simulink model "OMSv1_2"  (Simulink 6.6)
settings: Solver=ode4  SolverMode=SingleTasking  StartTime=0.0  StopTime=5  FixedStep=0.001  MaxStep=0.001  RelTol=1e-3  AbsTol=1e-3
undefined symbols (not defined in the file): alexlaw, bs_onoff, bs_scale, bsfsacrit, bsfsvcrit, cnsgain, fs_onoff, fs_scale, fsdelaycalc, ltdrk, phasicgain, pmcgain, pmctau2, pmctau3, saccsw, spgain, tonicgain, tvrD, tvrN
(part 3 of 7)

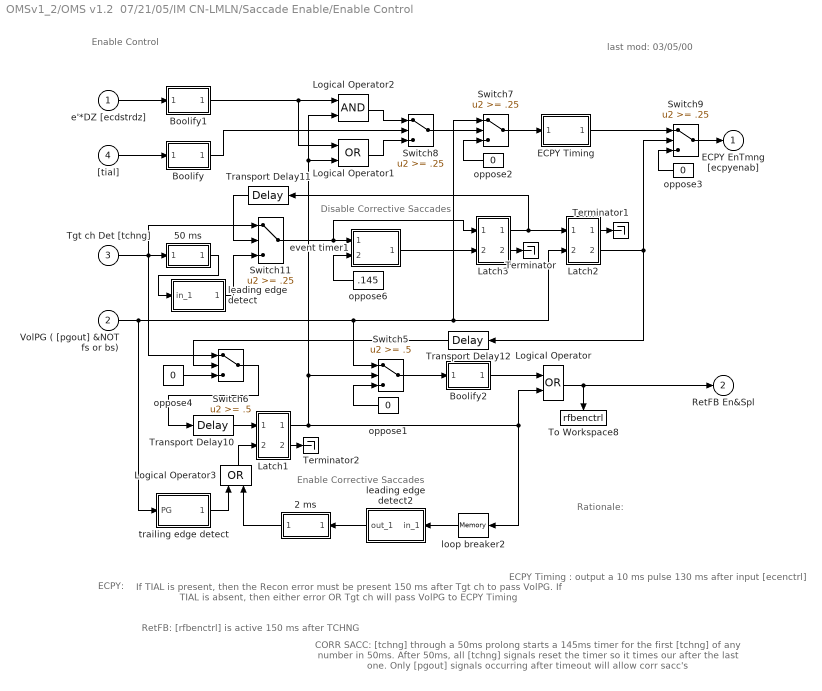
== system OMSv1_2/OMS v1.2  07/21/05/IM CN-LMLN/Saccade Enable/Enable Control ==
  note: Enable Control
  note: Enable
      | Corrective Saccades
  note: last mod:
      | 03/05/00
  note: Rationale:
  note: ECPY Timing : output a 10 ms pulse
      | 130 ms after input [ecenctrl]
  note: If TIAL is present, then the Recon error must be present 150 ms after Tgt ch to pass VolPG.
      | If TIAL is absent, then either error OR Tgt ch will pass VolPG to ECPY Timing
  note: ECPY:
  note: RetFB:
      | [rfbenctrl] is active 150 ms after TCHNG
  note: Disable
      | Corrective Saccades
  note: CORR SACC:
      | [tchng] through a 50ms prolong starts a 145ms timer for the
      | first [tchng] of any number in 50ms. After 50ms, all [tchng]
      | signals reset the timer so it times our after the last one.
      | Only [pgout] signals occurring after timeout will allow corr sacc's
  e'*DZ [ecdstrdz] : Inport
  VolPG ( [pgout] &NOT fs or bs) : Inport  Port=2
  Tgt ch Det [tchng] : Inport  Port=3
  "[tial]" : Inport  Port=4
  2 ms : Subsystem  Orientation=left  mask{prolong=2}
      mask prompts: prolong "Prolong pulse by?  (msec)"
      mask Display: disp('prolong')
  50 ms : Subsystem  mask{prolong=50}
      mask prompts: prolong "Prolong pulse by?  (msec)"
      mask Display: disp('prolong')
  Boolify : Subsystem
      mask Display: disp('Boolify')
  Boolify1 : Subsystem
      mask Display: disp('Boolify')
  Boolify2 : Subsystem
      mask Display: disp('Boolify')
  ECPY Timing : Subsystem
      mask Display: disp('ECPY\nTiming')
  Latch1 : Subsystem  mask(Latch){@1=0}
      mask prompts: @1 "Initial State for Output "Q":"
      mask help: Latch
      mask init:
      | ini=(@1~=0);
      mask Help: Latches the S input.  When S (set) is one, the Q output  becomes one.  The output remains one until the R (reset) input becomes one, forcing the output to zero.  If both R and S are one, the latch will be in an undefined state.
      mask Display: disp('S   Q\n\nR  !Q')
  Latch2 : Subsystem  mask(Latch){@1=0}
      mask prompts: @1 "Initial State for Output "Q":"
      mask help: Latch
      mask init:
      | ini=(@1~=0);
      mask Help: Latches the S input.  When S (set) is one, the Q output  becomes one.  The output remains one until the R (reset) input becomes one, forcing the output to zero.  If both R and S are one, the latch will be in an undefined state.
      mask Display: disp('S   Q\n\nR  !Q')
  Latch3 : Subsystem  mask(Latch){@1=0}
      mask prompts: @1 "Initial State for Output "Q":"
      mask help: Latch
      mask init:
      | ini=(@1~=0);
      mask Help: Latches the S input.  When S (set) is one, the Q output  becomes one.  The output remains one until the R (reset) input becomes one, forcing the output to zero.  If both R and S are one, the latch will be in an undefined state.
      mask Display: disp('S   Q\n\nR  !Q')
  Logical Operator : Logic  Operator=OR
  Logical Operator1 : Logic  Operator=OR
  Logical Operator2 : Logic
  Logical Operator3 : Logic  Orientation=up  Operator=OR
  Switch{7..9,11} (4 alike) : Switch  Threshold=.25  SaturateOnIntegerOverflow=on  InputSameDT=on
  Switch5 : Switch  Threshold=.5  SaturateOnIntegerOverflow=on  InputSameDT=on
  Switch6 : Switch  Threshold=.5  SaturateOnIntegerOverflow=on  InputSameDT=on
  Terminator : Terminator
  Terminator1 : Terminator
  Terminator2 : Terminator
  To Workspace8 : ToWorkspace  VariableName=rfbenctrl  SaveFormat=Array
      settings: Orientation=down  MaxDataPoints=10000
  Transport Delay10 : TransportDelay  DelayTime=.15
      mask Display: disp('150ms')
  Transport Delay11 : TransportDelay  Orientation=left  DelayTime=.05
      mask Display: disp('50ms')
  Transport Delay12 : TransportDelay  Orientation=left  DelayTime=.002
      mask Display: disp('2ms')
  event timer1 : Subsystem
      mask Display: disp('Event\nTimer2')
  leading edge detect : Subsystem
      mask Display: disp('Leading\nEdge Det')
  leading edge detect2 : Subsystem  Orientation=left
      mask Display: disp('Leading\nEdge Det')
  loop breaker2 : Memory  Orientation=left
  oppose1 : Constant  Orientation=left  Value=0
  oppose2 : Constant  Orientation=left  Value=0
  oppose3 : Constant  Orientation=left  Value=0
  oppose4 : Constant  Value=0
  oppose6 : Constant  Orientation=left  Value=.145
  trailing edge detect : Subsystem
      mask Display: disp('Trailing\nEdge Det')
  ECPY EnTmng [ecpyenab] : Outport  InitialOutput=0
  RetFB En&Spl : Outport  Port=2  InitialOutput=0
  wires:
  Boolify1/1(Out1) -> Logical Operator1/1, Logical Operator2/1
  "[tial]"/1 -> Boolify/1(In1)
  e'*DZ [ecdstrdz]/1 -> Boolify1/1(In1)
  Logical Operator1/1 -> Switch8/3
  Logical Operator2/1 -> Switch8/1
  Boolify/1(Out1) -> Switch8/2
  oppose2/1 -> Switch7/3
  Switch8/1 -> Switch7/2
  ECPY Timing/1(ECPY Enable [ecpyenab]) -> Switch9/1
  Switch9/1 -> ECPY EnTmng [ecpyenab]/1
  oppose3/1 -> Switch9/3
  Latch2/2(out_2) -> Transport Delay12/1, Switch9/2
  oppose6/1 -> event timer1/2(_timer value (port))
  Transport Delay11/1 -> Switch11/2
  Tgt ch Det [tchng]/1 -> 50 ms/1(value(in)), Switch6/1, Switch11/1
  Latch3/1(out_1) -> Latch2/1(in_1), Transport Delay11/1
  VolPG ( [pgout] &NOT fs or bs)/1 -> trailing edge detect/1(PG), Switch5/1, Switch7/1, Latch2/2(in_2)
  oppose1/1 -> Switch5/3
  Switch5/1 -> Boolify2/1(In1)
  Boolify2/1(Out1) -> Logical Operator/1
  Logical Operator/1 -> RetFB En&Spl/1, To Workspace8/1
  Latch1/1(out_1) -> Switch5/2, Logical Operator1/2, Logical Operator2/2, Logical Operator/2, loop breaker2/1
  Transport Delay10/1 -> Latch1/1(in_1)
  Logical Operator3/1 -> Latch1/2(in_2)
  oppose4/1 -> Switch6/3
  Switch6/1 -> Transport Delay10/1
  Transport Delay12/1 -> Switch6/2
  loop breaker2/1 -> leading edge detect2/1(in_1)
  50 ms/1(value(out)) -> leading edge detect/1(in_1)
  leading edge detect/1(out_1) -> Switch11/3
  Switch7/1 -> ECPY Timing/1(ECPY EnCntr [ecenctrl])
  event timer1/1(FF Reset) -> Latch3/2(in_2)
  Switch11/1 -> event timer1/1(SW out), Latch3/1(in_1)
  trailing edge detect/1(Latch R) -> Logical Operator3/1
  2 ms/1(value(out)) -> Logical Operator3/2
  leading edge detect2/1(out_1) -> 2 ms/1(value(in))
  Latch3/2(out_2) -> Terminator/1
  Latch2/1(out_1) -> Terminator1/1
  Latch1/2(out_2) -> Terminator2/1

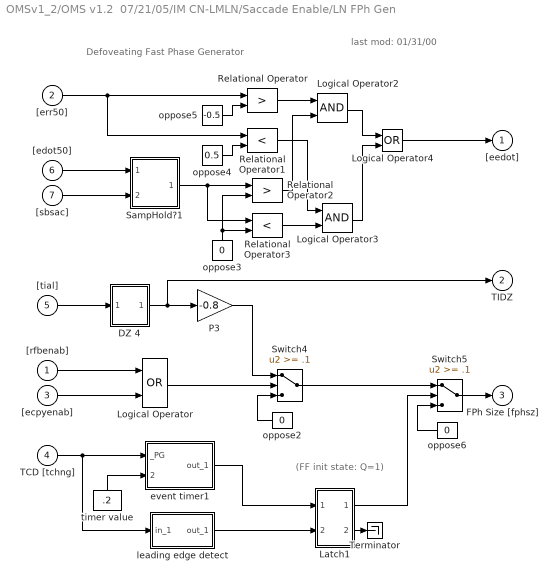
== system OMSv1_2/OMS v1.2  07/21/05/IM CN-LMLN/Saccade Enable/LN FPh Gen ==
  note: Defoveating Fast Phase Generator
  note: (FF init state: Q=1)
  note: last mod:
      | 01/31/00
  "[rfbenab]" : Inport
  "[err50]" : Inport  Port=2
  "[ecpyenab]" : Inport  Port=3
  TCD [tchng] : Inport  Port=4
  "[tial]" : Inport  Port=5
  "[edot50]" : Inport  Port=6
  "[sbsac]" : Inport  Port=7
  DZ 4 : Subsystem
      mask Display: disp('Dead\nZone')
  Latch1 : Subsystem  mask(Latch){@1=1}
      mask prompts: @1 "Initial State for Output "Q":"
      mask help: Latch
      mask init:
      | ini=(@1~=0);
      mask Help: Latches the S input.  When S (set) is one, the Q output  becomes one.  The output remains one until the R (reset) input becomes one, forcing the output to zero.  If both R and S are one, the latch will be in an undefined state.
      mask Display: disp('S   Q\n\nR  !Q')
  Logical Operator : Logic  Operator=OR
  Logical Operator2 : Logic
  Logical Operator3 : Logic
  Logical Operator4 : Logic  Operator=OR
  P3 : Gain  Gain=-0.8  SaturateOnIntegerOverflow=on
  Relational Operator : RelationalOperator  Operator=>  InputSameDT=on
  Relational Operator1 : RelationalOperator  Operator=<  InputSameDT=on
  Relational Operator2 : RelationalOperator  Operator=>  InputSameDT=on
  Relational Operator3 : RelationalOperator  Operator=<  InputSameDT=on
  SampHold?1 : Subsystem
      mask Display: disp('S&H\n(S=H)\n(H=L)')
  Switch4 : Switch  Threshold=.1  SaturateOnIntegerOverflow=on  InputSameDT=on
  Switch5 : Switch  Threshold=.1  SaturateOnIntegerOverflow=on  InputSameDT=on
  Terminator : Terminator
  event timer1 : Subsystem
      mask Display: disp('Event\nTimer2')
  leading edge detect : Subsystem
      mask Display: disp('Leading\nEdge Det')
  oppose2 : Constant  Orientation=left  Value=0
  oppose3 : Constant  Orientation=up  Value=0
  oppose4 : Constant  Value=0.5
  oppose5 : Constant  Value=-0.5
  oppose6 : Constant  Orientation=left  Value=0
  timer value : Constant  Orientation=up  Value=.2
  "[eedot]" : Outport  InitialOutput=0
  TIDZ : Outport  Port=2  InitialOutput=0
  FPh Size [fphsz] : Outport  Port=3  InitialOutput=0
  wires:
  "[err50]"/1 -> Relational Operator/1, Relational Operator1/1
  Logical Operator4/1 -> "[eedot]"/1
  Logical Operator2/1 -> Logical Operator4/1
  Relational Operator/1 -> Logical Operator2/1
  oppose5/1 -> Relational Operator/2
  oppose4/1 -> Relational Operator1/2
  Logical Operator3/1 -> Logical Operator4/2
  oppose3/1 -> Relational Operator3/2, Relational Operator2/2
  SampHold?1/1(output) -> Relational Operator2/1, Relational Operator3/1
  Relational Operator3/1 -> Logical Operator3/2
  Relational Operator2/1 -> Logical Operator2/2
  Relational Operator1/1 -> Logical Operator3/1
  "[sbsac]"/1 -> SampHold?1/2(S/H?)
  "[edot50]"/1 -> SampHold?1/1(Input)
  "[rfbenab]"/1 -> Logical Operator/1
  oppose2/1 -> Switch4/3
  "[ecpyenab]"/1 -> Logical Operator/2
  Switch4/1 -> Switch5/1
  Switch5/1 -> FPh Size [fphsz]/1
  oppose6/1 -> Switch5/3
  DZ 4/1(out_1) -> P3/1, TIDZ/1
  "[tial]"/1 -> DZ 4/1(in_1)
  event timer1/1(out_1) -> Latch1/1(in_1)
  leading edge detect/1(out_1) -> Latch1/2(in_2)
  Latch1/1(out_1) -> Switch5/2
  timer value/1 -> event timer1/2(_timer value (port))
  TCD [tchng]/1 -> event timer1/1(_PG), leading edge detect/1(in_1)
  P3/1 -> Switch4/1
  Logical Operator/1 -> Switch4/2
  Latch1/2(out_2) -> Terminator/1

== system OMSv1_2/OMS v1.2  07/21/05/IM CN-LMLN/Saccade Enable/Latch1 ==
  in_1 : Inport
  in_2 : Inport  Port=2
  Demux : Demux  Outputs=2
  Logic : CombinatorialLogic  TruthTable=[0 1;0 1;1 0;0 1;1 0;0 1;1 0;1 0]
  Memory : Memory  Orientation=left  X0=ini
  Mux : Mux  Inputs=3
  out_1 : Outport  InitialOutput=0
  out_2 : Outport  Port=2  InitialOutput=0
  wires:
  in_2/1 -> Mux/3
  in_1/1 -> Mux/2
  Memory/1 -> Mux/1
  Demux/1 -> Memory/1, out_1/1
  Mux/1 -> Logic/1
  Logic/1 -> Demux/1
  Demux/2 -> out_2/1

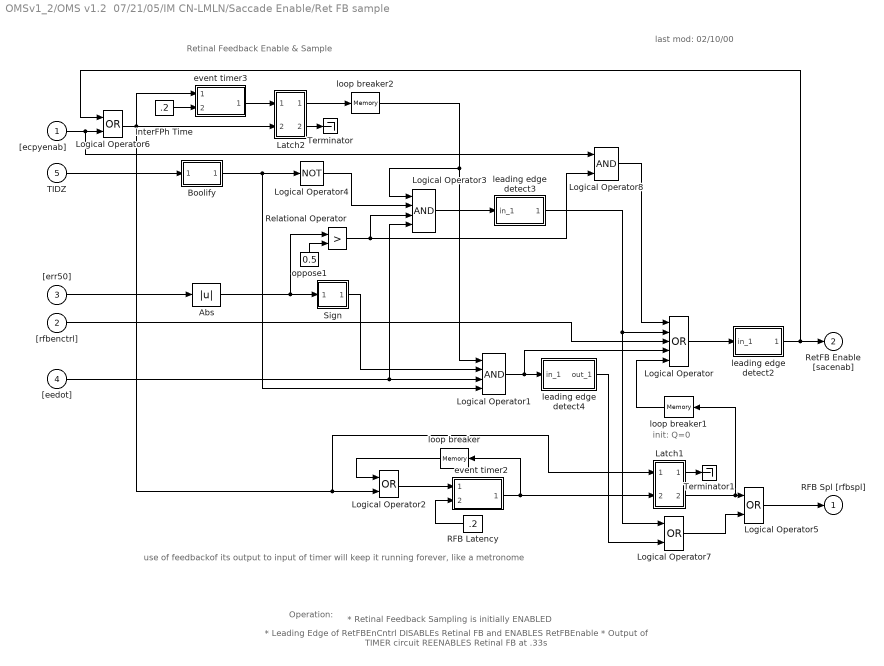
== system OMSv1_2/OMS v1.2  07/21/05/IM CN-LMLN/Saccade Enable/Ret FB sample ==
  note: * Leading Edge of RetFBEnCntrl DISABLEs Retinal FB
      |  and ENABLES RetFBEnable
      | * Output of TIMER circuit REENABLES Retinal FB at .33s
  note: * Retinal Feedback Sampling is initially ENABLED
  note: Operation:
  note: init: Q=0
  note: Retinal Feedback Enable & Sample
  note: last mod:
      | 02/10/00
  note: use of feedbackof its output to input of timer will
      | keep it running forever, like a metronome
  "[ecpyenab]" : Inport
  "[rfbenctrl]" : Inport  Port=2
  "[err50]" : Inport  Port=3
  "[eedot]" : Inport  Port=4
  TIDZ : Inport  Port=5
  Abs : Abs  SaturateOnIntegerOverflow=on
  Boolify : Subsystem
      mask Display: disp('Boolify')
  InterFPh Time : Constant  Value=.2
  Latch1 : Subsystem  mask(Latch){@1=0}
      mask prompts: @1 "Initial State for Output "Q":"
      mask help: Latch
      mask init:
      | ini=(@1~=0);
      mask Help: Latches the S input.  When S (set) is one, the Q output  becomes one.  The output remains one until the R (reset) input becomes one, forcing the output to zero.  If both R and S are one, the latch will be in an undefined state.
      mask Display: disp('S   Q\n\nR  !Q')
  Latch2 : Subsystem  mask(Latch){@1=1}
      mask prompts: @1 "Initial State for Output "Q":"
      mask help: Latch
      mask init:
      | ini=(@1~=0);
      mask Help: Latches the S input.  When S (set) is one, the Q output  becomes one.  The output remains one until the R (reset) input becomes one, forcing the output to zero.  If both R and S are one, the latch will be in an undefined state.
      mask Display: disp('S   Q\n\nR  !Q')
  Logical Operator : Logic  Operator=OR  Inputs=5
  Logical Operator1 : Logic  Inputs=4
  Logical Operator{2,5..7} (4 alike) : Logic  Operator=OR
  Logical Operator3 : Logic  Inputs=4
  Logical Operator4 : Logic  Operator=NOT  Inputs=1
  Logical Operator8 : Logic
  RFB Latency : Constant  Orientation=left  Value=.2
  Relational Operator : RelationalOperator  Operator=>  InputSameDT=on
  Sign : Subsystem
      mask Type: Sign
      mask Description: y = sign(x)
      mask Help: Sign Function:\n\t\t\ty = 1 if x > 0\n\t\t\ty = 0 if x = 0\n\t\t\ty = -1 if x < 0
      mask Display: plot(-50,-50,50,50,[-50,50],[0,0],[0,0],[-50,50],[-40,0],[-30,-30],[0,40],[30,30])
  Terminator : Terminator
  Terminator1 : Terminator
  event timer2 : Subsystem
      mask Display: disp('Event\nTimer2')
  event timer3 : Subsystem
      mask Display: disp('Event\nTimer2')
  leading edge detect2 : Subsystem
      mask Display: disp('Leading\nEdge Det')
  leading edge detect3 : Subsystem
      mask Display: disp('Leading\nEdge Det')
  leading edge detect4 : Subsystem
      mask Display: disp('Leading\nEdge Det')
  loop breaker : Memory  Orientation=left
  loop breaker1 : Memory  Orientation=left
  loop breaker2 : Memory
  oppose1 : Constant  Orientation=up  Value=0.5
  RFB Spl [rfbspl] : Outport  InitialOutput=0
  RetFB Enable [sacenab] : Outport  Port=2  InitialOutput=0
  wires:
  InterFPh Time/1 -> event timer3/2(_timer value (port))
  event timer3/1(outFF) -> Latch2/1(in_1)
  Latch2/1(out_1) -> loop breaker2/1
  Boolify/1(Out1) -> Logical Operator4/1, Logical Operator1/4
  TIDZ/1 -> Boolify/1(In1)
  loop breaker/1 -> Logical Operator2/1
  RFB Latency/1 -> event timer2/2(_timer value (port))
  oppose1/1 -> Relational Operator/2
  Abs/1 -> Sign/1(in_1), Relational Operator/1
  Logical Operator6/1 -> event timer3/1(RetFB EnCntrl), Latch2/2(in_2), Logical Operator2/2, Latch1/1(in_1)
  Logical Operator3/1 -> leading edge detect3/1(in_1)
  leading edge detect2/1(out_1) -> Logical Operator6/1, RetFB Enable [sacenab]/1
  Logical Operator1/1 -> leading edge detect4/1(in_1), Logical Operator/4
  leading edge detect4/1(out_1) -> Logical Operator7/2
  "[ecpyenab]"/1 -> Logical Operator6/2, Logical Operator8/1
  loop breaker1/1 -> Logical Operator/5
  "[rfbenctrl]"/1 -> Logical Operator/3
  leading edge detect3/1(out_1) -> Logical Operator7/1, Logical Operator/2
  event timer2/1(outFF) -> Latch1/2(in_2), loop breaker/1
  "[eedot]"/1 -> Logical Operator1/3, Logical Operator3/4
  Latch1/2(out_2) -> loop breaker1/1, Logical Operator5/1
  Logical Operator5/1 -> RFB Spl [rfbspl]/1
  Relational Operator/1 -> Logical Operator3/3, Logical Operator8/2
  Sign/1(out_1) -> Logical Operator1/2
  "[err50]"/1 -> Abs/1
  loop breaker2/1 -> Logical Operator1/1, Logical Operator3/1
  Logical Operator8/1 -> Logical Operator/1
  Logical Operator7/1 -> Logical Operator5/2
  Logical Operator2/1 -> event timer2/1(RetFB EnCntrl)
  Logical Operator4/1 -> Logical Operator3/2
  Logical Operator/1 -> leading edge detect2/1(in_1)
  Latch2/2(out_2) -> Terminator/1
  Latch1/1(out_1) -> Terminator1/1

== system OMSv1_2/OMS v1.2  07/21/05/IM CN-LMLN/Saccade Enable/leading edge detect2 ==
  note: It is also possible to remove the SIGNUM function
      | and the '==', and replace them with a simple
      | switch with a threshold of (say) 150 or so.
  note: leading edge detection
  in_1 : Inport
  Abs : Abs  SaturateOnIntegerOverflow=on
  Derivative : Derivative
  Relational Operator : RelationalOperator  Operator===  InputSameDT=on
  Sign : Subsystem
      mask Type: Sign
      mask Description: y = sign(x)
      mask Help: Sign Function:\n\t\t\ty = 1 if x > 0\n\t\t\ty = 0 if x = 0\n\t\t\ty = -1 if x < 0
      mask Display: plot(-50,-50,50,50,[-50,50],[0,0],[0,0],[-50,50],[-40,0],[-30,-30],[0,40],[30,30])
  Threshold 1 : Constant
  out_1 : Outport  InitialOutput=0
  wires:
  Abs/1 -> Derivative/1
  Derivative/1 -> Sign/1(in_1)
  Sign/1(out_1) -> Relational Operator/1
  Threshold 1/1 -> Relational Operator/2
  Relational Operator/1 -> out_1/1
  in_1/1 -> Abs/1

== system OMSv1_2/OMS v1.2  07/21/05/IM CN-LMLN/Saccade Enable/prolong ==
  note: init Q = 0
  note: Stretch the duration of an input pulse, latching it at its value at pulse onset.
  note: The one integration step delay before the S&H block's S/H (bottom) input insures
      | that the input value to be latched is available to theS&H block's top input
      | before the S&H block tries to 'hold'.
  note: The start of the input pulse causes the value on input 1 to be held starting when the leading
      | edge occurs, and this value remains latched until 'delay' seconds after the pulse ends (trailing edge).
  note: 11/22/99
  note: init = 0
  note: init = 0
  value(in) : Inport
  " x/1000" : Constant  Orientation=up  Value=0.001
  Latch1 : Subsystem  mask(Latch){@1=0}
      mask prompts: @1 "Initial State for Output "Q":"
      mask help: Latch
      mask init:
      | ini=(@1~=0);
      mask Help: Latches the S input.  When S (set) is one, the Q output  becomes one.  The output remains one until the R (reset) input becomes one, forcing the output to zero.  If both R and S are one, the latch will be in an undefined state.
      mask Display: disp('S   Q\n\nR  !Q')
  Product : Product  SaturateOnIntegerOverflow=on  RndMeth=Zero  InputSameDT=on
  SampHold?2 : Subsystem
      mask Display: disp('S=L\nH=H')
  Terminator : Terminator
  Variable Transport Delay : VariableTransportDelay  MaximumDelay=10  MaximumPoints=prolong_buffersize
  leading edge detect : Subsystem
      mask Display: disp('Leading\nEdge Det')
  loop breaker2 : Memory
  stretch : Constant  Value=prolong
  trailing edge detect : Subsystem
      mask Display: disp('Trailing\nEdge Det')
  value(out) : Outport  InitialOutput=0
  wires:
  value(in)/1 -> leading edge detect/1(in_1), trailing edge detect/1(in_1), SampHold?2/1(Input)
  Variable Transport Delay/1 -> Latch1/2(in_2)
  trailing edge detect/1(out_1) -> Variable Transport Delay/1
  leading edge detect/1(out_1) -> Latch1/1(in_1)
  Latch1/1(out_1) -> loop breaker2/1
  SampHold?2/1(output) -> value(out)/1
  loop breaker2/1 -> SampHold?2/2(S/H?)
  stretch/1 -> Product/1
  Product/1 -> Variable Transport Delay/2
  " x/1000"/1 -> Product/2
  Latch1/2(out_2) -> Terminator/1

== system OMSv1_2/OMS v1.2  07/21/05/IM CN-LMLN/Saccade Enable/trailing edge detect ==
  note: trailing edge detection
  note: It is also possible to remove the SIGNUM function
      | and the '==', and replace them with a simple
      | switch with a threshold of (say) 150 or so.
  PG : Inport
  Abs : Abs  SaturateOnIntegerOverflow=on
  Derivative : Derivative
  Relational Operator : RelationalOperator  Operator===  InputSameDT=on
  Sign : Subsystem
      mask Type: Sign
      mask Description: y = sign(x)
      mask Help: Sign Function:\n\t\t\ty = 1 if x > 0\n\t\t\ty = 0 if x = 0\n\t\t\ty = -1 if x < 0
      mask Display: plot(-50,-50,50,50,[-50,50],[0,0],[0,0],[-50,50],[-40,0],[-30,-30],[0,40],[30,30])
  Threshold 1 : Constant  Value=-1
  Latch R : Outport  InitialOutput=0
  wires:
  PG/1 -> Abs/1
  Relational Operator/1 -> Latch R/1
  Threshold 1/1 -> Relational Operator/2
  Sign/1(out_1) -> Relational Operator/1
  Derivative/1 -> Sign/1(in_1)
  Abs/1 -> Derivative/1

== system OMSv1_2/OMS v1.2  07/21/05/IM CN-LMLN/Saccade Motor Commmand/TCHNG Override ==
  note: (FF init state: Q=1)
  note: * Leading Edge of input ENABLEs output
  note: Operation:
  note: *FS Enabling is initially DISABLED
  note: * Output of TIMER circuit DISABLES output
  note: TCHNG Override
  "[tchng]" : Inport
  timer dur : Inport  Orientation=up  Port=2
  Latch1 : Subsystem  mask(Latch){@1=1}
      mask prompts: @1 "Initial State for Output "Q":"
      mask help: Latch
      mask init:
      | ini=(@1~=0);
      mask Help: Latches the S input.  When S (set) is one, the Q output  becomes one.  The output remains one until the R (reset) input becomes one, forcing the output to zero.  If both R and S are one, the latch will be in an undefined state.
      mask Display: disp('S   Q\n\nR  !Q')
  Terminator : Terminator
  event timer2 : Subsystem
      mask Display: disp('Event\nTimer2')
  leading edge detect : Subsystem
      mask Display: disp('Leading\nEdge Det')
  tchng sw : Outport  InitialOutput=0
  wires:
  "[tchng]"/1 -> leading edge detect/1(in_1), event timer2/1(_PG)
  timer dur/1 -> event timer2/2(_timer value (port))
  event timer2/1(out_1) -> Latch1/1(in_1)
  leading edge detect/1(out_1) -> Latch1/2(in_2)
  Latch1/1(out_1) -> tchng sw/1
  Latch1/2(out_2) -> Terminator/1

== system OMSv1_2/OMS v1.2  07/21/05/IM CN-LMLN/Saccade Motor Commmand/Voluntary Saccade Switch ==
  note: Voluntary Saccade Switch
  note: move this outpt
      | to top switch
  note: last mod:
      | 02/26/01
  "[fphmag]" : Inport
  "[sacenab]" : Inport  Port=2
  "[fsorbs30]" : Inport  Port=3
  (0.5)1 : Switch  Threshold=.5  SaturateOnIntegerOverflow=on  InputSameDT=on
  (0.5)2 : Switch  Threshold=.5  SaturateOnIntegerOverflow=on  InputSameDT=on
  (0.5)3 : Switch  Threshold=.5  SaturateOnIntegerOverflow=on  InputSameDT=on
  Logical Operator4 : Logic  Operator=NOT  Inputs=1
  Logical Operator6 : Logic  Operator=OR
  oppose3 : Constant  Orientation=left  Value=0
  saccsw : Constant  Orientation=left  Value=saccsw
  "[vsmc]" : Outport  InitialOutput=0
  sacenab/0 : Outport  Port=2  InitialOutput=0
  wires:
  "[fphmag]"/1 -> (0.5)2/1
  "[fsorbs30]"/1 -> Logical Operator4/1
  Logical Operator4/1 -> Logical Operator6/2
  (0.5)2/1 -> (0.5)3/1
  Logical Operator6/1 -> sacenab/0/1
  saccsw/1 -> (0.5)2/3, (0.5)2/2, (0.5)1/2, (0.5)1/3
  "[sacenab]"/1 -> (0.5)1/1, (0.5)3/2
  (0.5)1/1 -> Logical Operator6/1
  oppose3/1 -> (0.5)3/3
  (0.5)3/1 -> "[vsmc]"/1

== system OMSv1_2/OMS v1.2  07/21/05/IM CN-LMLN/Sampled Target Reconstruction/Boolify ==
  In1 : Inport
  Abs2 : Abs  SaturateOnIntegerOverflow=on
  direction1 : Subsystem
      mask Type: Sign
      mask Description: y = sign(x)
      mask Help: Sign Function:\n\t\t\ty = 1 if x > 0\n\t\t\ty = 0 if x = 0\n\t\t\ty = -1 if x < 0
      mask Display: plot(-50,-50,50,50,[-50,50],[0,0],[0,0],[-50,50],[-40,0],[-30,-30],[0,40],[30,30])
  Out1 : Outport  InitialOutput=0
  wires:
  direction1/1(out_1) -> Out1/1
  In1/1 -> Abs2/1
  Abs2/1 -> direction1/1(in_1)

== system OMSv1_2/OMS v1.2  07/21/05/IM CN-LMLN/Sampled Target Reconstruction/Boolify1 ==
  In1 : Inport
  Abs2 : Abs  SaturateOnIntegerOverflow=on
  direction1 : Subsystem
      mask Type: Sign
      mask Description: y = sign(x)
      mask Help: Sign Function:\n\t\t\ty = 1 if x > 0\n\t\t\ty = 0 if x = 0\n\t\t\ty = -1 if x < 0
      mask Display: plot(-50,-50,50,50,[-50,50],[0,0],[0,0],[-50,50],[-40,0],[-30,-30],[0,40],[30,30])
  Out1 : Outport  InitialOutput=0
  wires:
  Abs2/1 -> direction1/1(in_1)
  In1/1 -> Abs2/1
  direction1/1(out_1) -> Out1/1

== system OMSv1_2/OMS v1.2  07/21/05/IM CN-LMLN/Sampled Target Reconstruction/DZ 0.3 ==
  note: We just output zero when the dead zone is in effect, and leave the
      |  output alone the rest of the time.
  note: This block is a better implementation of a dead zone than  the
      | block supplied by SIMULINK, because here we don't _subtract_
      | the dead zone from the rest of output.
  in_1 : Inport
  Abs : Abs  Orientation=down  SaturateOnIntegerOverflow=on
  Relational Operator : RelationalOperator  InputSameDT=on
  Switch6 : Switch  Threshold=.5  SaturateOnIntegerOverflow=on  InputSameDT=on
  dead zone : Constant  Orientation=up  Value=.3
  pos (deg) criterion1 : Constant  Orientation=left  Value=0
  out_1 : Outport  InitialOutput=0
  wires:
  Relational Operator/1 -> Switch6/2
  dead zone/1 -> Relational Operator/2
  pos (deg) criterion1/1 -> Switch6/3
  Abs/1 -> Relational Operator/1
  in_1/1 -> Abs/1, Switch6/1
  Switch6/1 -> out_1/1

== system OMSv1_2/OMS v1.2  07/21/05/IM CN-LMLN/Sampled Target Reconstruction/Latch1 ==
  in_1 : Inport
  in_2 : Inport  Port=2
  Demux : Demux  Outputs=2
  Logic : CombinatorialLogic  TruthTable=[0 1;0 1;1 0;0 1;1 0;0 1;1 0;1 0]
  Memory : Memory  Orientation=left  X0=ini
  Mux : Mux  Inputs=3
  out_1 : Outport  InitialOutput=0
  out_2 : Outport  Port=2  InitialOutput=0
  wires:
  in_2/1 -> Mux/3
  in_1/1 -> Mux/2
  Memory/1 -> Mux/1
  Demux/1 -> out_1/1, Memory/1
  Mux/1 -> Logic/1
  Logic/1 -> Demux/1
  Demux/2 -> out_2/1

== system OMSv1_2/OMS v1.2  07/21/05/IM CN-LMLN/Sampled Target Reconstruction/Latch2 ==
  in_1 : Inport
  in_2 : Inport  Port=2
  Demux : Demux  Outputs=2
  Logic : CombinatorialLogic  TruthTable=[0 1;0 1;1 0;0 1;1 0;0 1;1 0;1 0]
  Memory : Memory  Orientation=left  X0=ini
  Mux : Mux  Inputs=3
  out_1 : Outport  InitialOutput=0
  out_2 : Outport  Port=2  InitialOutput=0
  wires:
  Demux/2 -> out_2/1
  Logic/1 -> Demux/1
  Mux/1 -> Logic/1
  Demux/1 -> Memory/1, out_1/1
  Memory/1 -> Mux/1
  in_1/1 -> Mux/2
  in_2/1 -> Mux/3

== system OMSv1_2/OMS v1.2  07/21/05/IM CN-LMLN/Sampled Target Reconstruction/SampHold? ==
  note: When "S/H?" is HIGH, then "Input" is switched directly to the
      | output ("sample").  When "S/H?" is LOW, the current output is
      | maintained ("hold").
  Input : Inport
  S/H? : Inport  Port=2
  Memory : Memory  Orientation=left
  Sign : Subsystem
      mask Type: Sign
      mask Description: y = sign(x)
      mask Help: Sign Function:\n\t\t\ty = 1 if x > 0\n\t\t\ty = 0 if x = 0\n\t\t\ty = -1 if x < 0
      mask Display: plot(-50,-50,50,50,[-50,50],[0,0],[0,0],[-50,50],[-40,0],[-30,-30],[0,40],[30,30])
  Switch2 : Switch  Threshold=0.5  SaturateOnIntegerOverflow=on  InputSameDT=on
  output : Outport  InitialOutput=0
  wires:
  S/H?/1 -> Sign/1(in_1)
  Sign/1(out_1) -> Switch2/2
  Input/1 -> Switch2/1
  Switch2/1 -> output/1, Memory/1
  Memory/1 -> Switch2/3

== system OMSv1_2/OMS v1.2  07/21/05/IM CN-LMLN/Sampled Target Reconstruction/leading edge detect1 ==
  note: leading edge detection
  in_1 : Inport
  Abs : Abs  SaturateOnIntegerOverflow=on
  Derivative : Derivative
  Relational Operator : RelationalOperator  Operator===  InputSameDT=on
  Sign : Subsystem
      mask Type: Sign
      mask Description: y = sign(x)
      mask Help: Sign Function:\n\t\t\ty = 1 if x > 0\n\t\t\ty = 0 if x = 0\n\t\t\ty = -1 if x < 0
      mask Display: plot(-50,-50,50,50,[-50,50],[0,0],[0,0],[-50,50],[-40,0],[-30,-30],[0,40],[30,30])
  Threshold 1 : Constant
  out_1 : Outport  InitialOutput=0
  wires:
  Abs/1 -> Derivative/1
  Derivative/1 -> Sign/1(in_1)
  Sign/1(out_1) -> Relational Operator/1
  Threshold 1/1 -> Relational Operator/2
  Relational Operator/1 -> out_1/1
  in_1/1 -> Abs/1

== system OMSv1_2/OMS v1.2  07/21/05/IM CN-LMLN/Sampled Target Reconstruction/leading edge detect2 ==
  note: leading edge detection
  in_1 : Inport
  Abs : Abs  SaturateOnIntegerOverflow=on
  Derivative : Derivative
  Relational Operator : RelationalOperator  Operator===  InputSameDT=on
  Sign : Subsystem
      mask Type: Sign
      mask Description: y = sign(x)
      mask Help: Sign Function:\n\t\t\ty = 1 if x > 0\n\t\t\ty = 0 if x = 0\n\t\t\ty = -1 if x < 0
      mask Display: plot(-50,-50,50,50,[-50,50],[0,0],[0,0],[-50,50],[-40,0],[-30,-30],[0,40],[30,30])
  Threshold 1 : Constant
  out_1 : Outport  InitialOutput=0
  wires:
  in_1/1 -> Abs/1
  Relational Operator/1 -> out_1/1
  Threshold 1/1 -> Relational Operator/2
  Sign/1(out_1) -> Relational Operator/1
  Derivative/1 -> Sign/1(in_1)
  Abs/1 -> Derivative/1

== system OMSv1_2/OMS v1.2  07/21/05/IM CN-LMLN/Sampled Target Reconstruction/prolong ==
  note: init = 0
  note: init = 0
  note: 11/22/99
  note: The start of the input pulse causes the value on input 1 to be held starting when the leading
      | edge occurs, and this value remains latched until 'delay' seconds after the pulse ends (trailing edge).
  note: The one integration step delay before the S&H block's S/H (bottom) input insures
      | that the input value to be latched is available to theS&H block's top input
      | before the S&H block tries to 'hold'.
  note: Stretch the duration of an input pulse, latching it at its value at pulse onset.
  note: init Q = 0
  value(in) : Inport
  " x/1000" : Constant  Orientation=up  Value=0.001
  Latch1 : Subsystem  mask(Latch){@1=0}
      mask prompts: @1 "Initial State for Output "Q":"
      mask help: Latch
      mask init:
      | ini=(@1~=0);
      mask Help: Latches the S input.  When S (set) is one, the Q output  becomes one.  The output remains one until the R (reset) input becomes one, forcing the output to zero.  If both R and S are one, the latch will be in an undefined state.
      mask Display: disp('S   Q\n\nR  !Q')
  Product : Product  SaturateOnIntegerOverflow=on  RndMeth=Zero  InputSameDT=on
  SampHold?2 : Subsystem
      mask Display: disp('S=L\nH=H')
  Terminator : Terminator
  Variable Transport Delay : VariableTransportDelay  MaximumDelay=10  MaximumPoints=prolong_buffersize
  leading edge detect : Subsystem
      mask Display: disp('Leading\nEdge Det')
  loop breaker2 : Memory
  stretch : Constant  Value=prolong
  trailing edge detect : Subsystem
      mask Display: disp('Trailing\nEdge Det')
  value(out) : Outport  InitialOutput=0
  wires:
  " x/1000"/1 -> Product/2
  Product/1 -> Variable Transport Delay/2
  stretch/1 -> Product/1
  loop breaker2/1 -> SampHold?2/2(S/H?)
  SampHold?2/1(output) -> value(out)/1
  Latch1/1(out_1) -> loop breaker2/1
  leading edge detect/1(out_1) -> Latch1/1(in_1)
  trailing edge detect/1(out_1) -> Variable Transport Delay/1
  Variable Transport Delay/1 -> Latch1/2(in_2)
  value(in)/1 -> SampHold?2/1(Input), trailing edge detect/1(in_1), leading edge detect/1(in_1)
  Latch1/2(out_2) -> Terminator/1

== system OMSv1_2/OMS v1.2  07/21/05/IM CN-LMLN/Sampled Target Reconstruction/prolong1 ==
  note: init Q = 0
  note: Stretch the duration of an input pulse, latching it at its value at pulse onset.
  note: The one integration step delay before the S&H block's S/H (bottom) input insures
      | that the input value to be latched is available to theS&H block's top input
      | before the S&H block tries to 'hold'.
  note: The start of the input pulse causes the value on input 1 to be held starting when the leading
      | edge occurs, and this value remains latched until 'delay' seconds after the pulse ends (trailing edge).
  note: 11/22/99
  note: init = 0
  note: init = 0
  value(in) : Inport
  " x/1000" : Constant  Orientation=up  Value=0.001
  Latch1 : Subsystem  mask(Latch){@1=0}
      mask prompts: @1 "Initial State for Output "Q":"
      mask help: Latch
      mask init:
      | ini=(@1~=0);
      mask Help: Latches the S input.  When S (set) is one, the Q output  becomes one.  The output remains one until the R (reset) input becomes one, forcing the output to zero.  If both R and S are one, the latch will be in an undefined state.
      mask Display: disp('S   Q\n\nR  !Q')
  Product : Product  SaturateOnIntegerOverflow=on  RndMeth=Zero  InputSameDT=on
  SampHold?2 : Subsystem
      mask Display: disp('S=L\nH=H')
  Terminator : Terminator
  Variable Transport Delay : VariableTransportDelay  MaximumDelay=10  MaximumPoints=prolong_buffersize
  leading edge detect : Subsystem
      mask Display: disp('Leading\nEdge Det')
  loop breaker2 : Memory
  stretch : Constant  Value=prolong
  trailing edge detect : Subsystem
      mask Display: disp('Trailing\nEdge Det')
  value(out) : Outport  InitialOutput=0
  wires:
  value(in)/1 -> leading edge detect/1(in_1), trailing edge detect/1(in_1), SampHold?2/1(Input)
  Variable Transport Delay/1 -> Latch1/2(in_2)
  trailing edge detect/1(out_1) -> Variable Transport Delay/1
  leading edge detect/1(out_1) -> Latch1/1(in_1)
  Latch1/1(out_1) -> loop breaker2/1
  SampHold?2/1(output) -> value(out)/1
  loop breaker2/1 -> SampHold?2/2(S/H?)
  stretch/1 -> Product/1
  Product/1 -> Variable Transport Delay/2
  " x/1000"/1 -> Product/2
  Latch1/2(out_2) -> Terminator/1

== system OMSv1_2/OMS v1.2  07/21/05/IM CN-LMLN/Sampled Target Reconstruction/prolong2 ==
  note: init = 0
  note: init = 0
  note: 11/22/99
  note: The start of the input pulse causes the value on input 1 to be held starting when the leading
      | edge occurs, and this value remains latched until 'delay' seconds after the pulse ends (trailing edge).
  note: The one integration step delay before the S&H block's S/H (bottom) input insures
      | that the input value to be latched is available to theS&H block's top input
      | before the S&H block tries to 'hold'.
  note: Stretch the duration of an input pulse, latching it at its value at pulse onset.
  note: init Q = 0
  value(in) : Inport
  " x/1000" : Constant  Orientation=up  Value=0.001
  Latch1 : Subsystem  mask(Latch){@1=0}
      mask prompts: @1 "Initial State for Output "Q":"
      mask help: Latch
      mask init:
      | ini=(@1~=0);
      mask Help: Latches the S input.  When S (set) is one, the Q output  becomes one.  The output remains one until the R (reset) input becomes one, forcing the output to zero.  If both R and S are one, the latch will be in an undefined state.
      mask Display: disp('S   Q\n\nR  !Q')
  Product : Product  SaturateOnIntegerOverflow=on  RndMeth=Zero  InputSameDT=on
  SampHold?2 : Subsystem
      mask Display: disp('S=L\nH=H')
  Terminator : Terminator
  Variable Transport Delay : VariableTransportDelay  MaximumDelay=10  MaximumPoints=prolong_buffersize
  leading edge detect : Subsystem
      mask Display: disp('Leading\nEdge Det')
  loop breaker2 : Memory
  stretch : Constant  Value=prolong
  trailing edge detect : Subsystem
      mask Display: disp('Trailing\nEdge Det')
  value(out) : Outport  InitialOutput=0
  wires:
  " x/1000"/1 -> Product/2
  Product/1 -> Variable Transport Delay/2
  stretch/1 -> Product/1
  loop breaker2/1 -> SampHold?2/2(S/H?)
  SampHold?2/1(output) -> value(out)/1
  Latch1/1(out_1) -> loop breaker2/1
  leading edge detect/1(out_1) -> Latch1/1(in_1)
  trailing edge detect/1(out_1) -> Variable Transport Delay/1
  Variable Transport Delay/1 -> Latch1/2(in_2)
  value(in)/1 -> SampHold?2/1(Input), trailing edge detect/1(in_1), leading edge detect/1(in_1)
  Latch1/2(out_2) -> Terminator/1

== system OMSv1_2/OMS v1.2  07/21/05/IM CN-LMLN/Slip Velocity Reconstruction/DZ 0.5 ==
  note: We just output zero when the dead zone is in effect, and leave the
      |  output alone the rest of the time.
  note: This block is a better implementation of a dead zone than  the
      | block supplied by SIMULINK, because here we don't _subtract_
      | the dead zone from the rest of output.
  in_1 : Inport
  in_2 : Inport  Port=2
  Abs : Abs  Orientation=down  SaturateOnIntegerOverflow=on
  Relational Operator : RelationalOperator  InputSameDT=on
  Switch6 : Switch  Threshold=.5  SaturateOnIntegerOverflow=on  InputSameDT=on
  pos (deg) criterion1 : Constant  Orientation=left  Value=0
  out_1 : Outport  InitialOutput=0
  wires:
  Relational Operator/1 -> Switch6/2
  pos (deg) criterion1/1 -> Switch6/3
  Switch6/1 -> out_1/1
  in_2/1 -> Relational Operator/2
  Abs/1 -> Relational Operator/1
  in_1/1 -> Abs/1, Switch6/1

== system OMSv1_2/OMS v1.2  07/21/05/IM CN-LMLN/Slip Velocity Reconstruction/Lim 100 ==
  note: This block limits outputs to less than or equal to the "Limit" constant.
      | Inputs greater than "Limit" yield a zero output.
  in_1 : Inport
  Abs : Abs  SaturateOnIntegerOverflow=on
  Limit : Constant  Orientation=up  Value=100
  Product : Product  SaturateOnIntegerOverflow=on  RndMeth=Zero  InputSameDT=on
  Relational Operator : RelationalOperator  Operator=<=  InputSameDT=on
  out_1 : Outport  InitialOutput=0
  wires:
  in_1/1 -> Product/1, Abs/1
  Abs/1 -> Relational Operator/1
  Relational Operator/1 -> Product/2
  Limit/1 -> Relational Operator/2
  Product/1 -> out_1/1

== system OMSv1_2/OMS v1.2  07/21/05/IM CN-LMLN/Slip Velocity Reconstruction/SampHold?4 ==
  note: When "S/H?" is HIGH, then "Input" is switched directly to the
      | output ("sample").  When "S/H?" is LOW, the current output is
      | maintained ("hold").
  Input : Inport
  S/H? : Inport  Port=2
  Memory : Memory  Orientation=left
  Sign : Subsystem
      mask Type: Sign
      mask Description: y = sign(x)
      mask Help: Sign Function:\n\t\t\ty = 1 if x > 0\n\t\t\ty = 0 if x = 0\n\t\t\ty = -1 if x < 0
      mask Display: plot(-50,-50,50,50,[-50,50],[0,0],[0,0],[-50,50],[-40,0],[-30,-30],[0,40],[30,30])
  Switch2 : Switch  Threshold=0.5  SaturateOnIntegerOverflow=on  InputSameDT=on
  output : Outport  InitialOutput=0
  wires:
  S/H?/1 -> Sign/1(in_1)
  Sign/1(out_1) -> Switch2/2
  Switch2/1 -> output/1, Memory/1
  Input/1 -> Switch2/1
  Memory/1 -> Switch2/3

== system OMSv1_2/OMS v1.2  07/21/05/OMN2/SampHold?/Sign ==
  in_1 : Inport
  Constant : Constant  Value=0
  Relational Operator : RelationalOperator  Operator=>  InputSameDT=on
  Relational Operator1 : RelationalOperator  Operator=<  InputSameDT=on
  Sum : Sum  Inputs=+-  SaturateOnIntegerOverflow=on  InputSameDT=on
  out_1 : Outport  InitialOutput=0
  wires:
  in_1/1 -> Relational Operator/1, Relational Operator1/1
  Constant/1 -> Relational Operator1/2, Relational Operator/2
  Relational Operator1/1 -> Sum/2
  Relational Operator/1 -> Sum/1
  Sum/1 -> out_1/1

== system OMSv1_2/OMS v1.2  07/21/05/PG w rNI1/PW funct/Good Reset Integrator1 ==
  note: This Resettable integrator won't (incorrectly) integrate the input even
      | when the reset signal is held, unlike the SIMULINK RI, which
      | gives a one time-step error.
  input : Inport
  reset? : Inport  Port=2
  initial condition : Inport  Port=3
  Logical Operator2 : Logic  Orientation=up  Operator=NOT  Inputs=1
  Product : Product  SaturateOnIntegerOverflow=on  RndMeth=Zero  InputSameDT=on
  Reset Integrator : ResetIntegrator
  out_1 : Outport  InitialOutput=0
  wires:
  initial condition/1 -> Reset Integrator/3
  Logical Operator2/1 -> Product/2
  input/1 -> Product/1
  Product/1 -> Reset Integrator/1
  reset?/1 -> Logical Operator2/1, Reset Integrator/2
  Reset Integrator/1 -> out_1/1

== system OMSv1_2/OMS v1.2  07/21/05/PG w rNI1/PW funct/Input Switch ==
  mcspl : Inport
  pgw : Inport  Port=2
  Switch2 : Switch  Threshold=0.5  SaturateOnIntegerOverflow=on  InputSameDT=on
  lead/trail edge det : Subsystem
      mask Display: disp('Lead/Trail\nEdge Det')
  mcsw : Outport  InitialOutput=0
  wires:
  mcspl/1 -> Switch2/1, lead/trail edge det/1(in_1)
  pgw/1 -> Switch2/2
  lead/trail edge det/1(out_1) -> Switch2/3
  Switch2/1 -> mcsw/1

== system OMSv1_2/OMS v1.2  07/21/05/PG w rNI1/PW funct/Sign ==
  in_1 : Inport
  Constant : Constant  Value=0
  Relational Operator : RelationalOperator  Operator=>  InputSameDT=on
  Relational Operator1 : RelationalOperator  Operator=<  InputSameDT=on
  Sum : Sum  Inputs=+-  SaturateOnIntegerOverflow=on  InputSameDT=on
  out_1 : Outport  InitialOutput=0
  wires:
  Sum/1 -> out_1/1
  Relational Operator/1 -> Sum/1
  Relational Operator1/1 -> Sum/2
  Constant/1 -> Relational Operator1/2, Relational Operator/2
  in_1/1 -> Relational Operator/1, Relational Operator1/1

== system OMSv1_2/OMS v1.2  07/21/05/PG w rNI1/RefLatch (Default = 50ms)/trailing edge ==
  note: (FF init state: Q=1)
  note: (Init input: 0)
  note: When the latency period is over, the block is again ENABLED.  ONLY once the latency period is
      | over does the block accept any new input.  (i.e. any input that occurs during the disabled
      |  latency period is ignored)
  note: When input occurs, the block then becomes DISABLED, and remains so for the
      | duration of the latency period (set either via the mask, or by setting "delay" from the command line)
  note: Block operation: it is initially ENABLED, allowing input.
  note: latency period starts with the END of the pulse, rather than the beginning.
  note: (Init input: 1)
  note: (Must see a trailing edge from the
      | signal AS WELL)
  note: This upper branch prevents response
      | to transients caused by the switch
      | toggling states
  in_1 : Inport
  Logical Operator : Logic
  S-R Flip-Flop : Subsystem  mask(Latch){@1=1}
      mask prompts: @1 "Initial State for Output "Q":"
      mask help: Latch
      mask init:
      | ini=(@1~=0);
      mask Help: Latches the S input.  When S (set) is one, the Q output  becomes one.  The output remains one until the R (reset) input becomes one, forcing the output to zero.  If both R and S are one, the latch will be in an undefined state.
      mask Display: disp('S   Q\n\nR  !Q')
  Switch1 : Switch  Threshold=.5  SaturateOnIntegerOverflow=on  InputSameDT=on
  Terminator : Terminator
  Threshold 3 : Constant  Orientation=left  Value=0
  loop breaker : Memory  Orientation=left  X0=1
  refractory period : TransportDelay  DelayTime=(delay)/1000
  trailing edge det : Subsystem
      mask Display: disp('Trailing\nEdge Det')
  trailing edge det1 : Subsystem
      mask Display: disp('Trailing\nEdge Det')
  out_1 : Outport  InitialOutput=0
  wires:
  S-R Flip-Flop/1(out_1) -> out_1/1, loop breaker/1
  Logical Operator/1 -> S-R Flip-Flop/2(in_2), refractory period/1
  trailing edge det/1(out_1) -> Logical Operator/1
  trailing edge det1/1(out_1) -> Logical Operator/2
  in_1/1 -> Switch1/1, trailing edge det/1(in_1)
  refractory period/1 -> S-R Flip-Flop/1(in_1)
  loop breaker/1 -> Switch1/2
  Threshold 3/1 -> Switch1/3
  Switch1/1 -> trailing edge det1/1(in_1)
  S-R Flip-Flop/2(out_2) -> Terminator/1

== system OMSv1_2/OMS v1.2  07/21/05/PG w rNI1/SampHold?1/Sign ==
  in_1 : Inport
  Constant : Constant  Value=0
  Relational Operator : RelationalOperator  Operator=>  InputSameDT=on
  Relational Operator1 : RelationalOperator  Operator=<  InputSameDT=on
  Sum : Sum  Inputs=+-  SaturateOnIntegerOverflow=on  InputSameDT=on
  out_1 : Outport  InitialOutput=0
  wires:
  Sum/1 -> out_1/1
  Relational Operator/1 -> Sum/1
  Relational Operator1/1 -> Sum/2
  Constant/1 -> Relational Operator1/2, Relational Operator/2
  in_1/1 -> Relational Operator/1, Relational Operator1/1

== system OMSv1_2/OMS v1.2  07/21/05/Fixation/30 /SampHold?2/Sign ==
  in_1 : Inport
  Constant : Constant  Value=0
  Relational Operator : RelationalOperator  Operator=>  InputSameDT=on
  Relational Operator1 : RelationalOperator  Operator=<  InputSameDT=on
  Sum : Sum  Inputs=+-  SaturateOnIntegerOverflow=on  InputSameDT=on
  out_1 : Outport  InitialOutput=0
  wires:
  in_1/1 -> Relational Operator/1, Relational Operator1/1
  Constant/1 -> Relational Operator1/2, Relational Operator/2
  Relational Operator1/1 -> Sum/2
  Relational Operator/1 -> Sum/1
  Sum/1 -> out_1/1

== system OMSv1_2/OMS v1.2  07/21/05/Fixation/30 /leading edge detect/Sign ==
  in_1 : Inport
  Constant : Constant  Value=0
  Relational Operator : RelationalOperator  Operator=>  InputSameDT=on
  Relational Operator1 : RelationalOperator  Operator=<  InputSameDT=on
  Sum : Sum  Inputs=+-  SaturateOnIntegerOverflow=on  InputSameDT=on
  out_1 : Outport  InitialOutput=0
  wires:
  Sum/1 -> out_1/1
  Relational Operator/1 -> Sum/1
  Relational Operator1/1 -> Sum/2
  Constant/1 -> Relational Operator/2, Relational Operator1/2
  in_1/1 -> Relational Operator1/1, Relational Operator/1

== system OMSv1_2/OMS v1.2  07/21/05/Fixation/30 /trailing edge detect/Sign ==
  in_1 : Inport
  Constant : Constant  Value=0
  Relational Operator : RelationalOperator  Operator=>  InputSameDT=on
  Relational Operator1 : RelationalOperator  Operator=<  InputSameDT=on
  Sum : Sum  Inputs=+-  SaturateOnIntegerOverflow=on  InputSameDT=on
  out_1 : Outport  InitialOutput=0
  wires:
  in_1/1 -> Relational Operator/1, Relational Operator1/1
  Constant/1 -> Relational Operator1/2, Relational Operator/2
  Relational Operator1/1 -> Sum/2
  Relational Operator/1 -> Sum/1
  Sum/1 -> out_1/1

== system OMSv1_2/OMS v1.2  07/21/05/IM CN-LMLN/Alexander's Law/Boolify/direction1 ==
  in_1 : Inport
  Constant : Constant  Value=0
  Relational Operator : RelationalOperator  Operator=>  InputSameDT=on
  Relational Operator1 : RelationalOperator  Operator=<  InputSameDT=on
  Sum : Sum  Inputs=+-  SaturateOnIntegerOverflow=on  InputSameDT=on
  out_1 : Outport  InitialOutput=0
  wires:
  Sum/1 -> out_1/1
  Relational Operator/1 -> Sum/1
  Relational Operator1/1 -> Sum/2
  Constant/1 -> Relational Operator/2, Relational Operator1/2
  in_1/1 -> Relational Operator1/1, Relational Operator/1

== system OMSv1_2/OMS v1.2  07/21/05/IM CN-LMLN/BS/FS Logic/BS Enable1/BS Timing ==
  note: (FF init state: Q=0)
  note: * Leading Edge of input ENABLEs output
  note: Operation:
  note: *BS Enabling is initially DISABLED
  note: * Output of TIMER circuit DISABLES output
  note: BS Timing
  From  <= [cmpr] : Inport
  timer dur : Inport  Orientation=up  Port=2
  Latch1 : Subsystem  mask(Latch){@1=0}
      mask prompts: @1 "Initial State for Output "Q":"
      mask help: Latch
      mask init:
      | ini=(@1~=0);
      mask Help: Latches the S input.  When S (set) is one, the Q output  becomes one.  The output remains one until the R (reset) input becomes one, forcing the output to zero.  If both R and S are one, the latch will be in an undefined state.
      mask Display: disp('S   Q\n\nR  !Q')
  Terminator : Terminator
  event timer2 : Subsystem
      mask Display: disp('Event\nTimer2')
  leading edge detect : Subsystem
      mask Display: disp('Leading\nEdge Det')
  "[bsenab]" : Outport  InitialOutput=0
  wires:
  From  <= [cmpr]/1 -> leading edge detect/1(in_1), event timer2/1(_PG)
  leading edge detect/1(out_1) -> Latch1/1(in_1)
  event timer2/1(out_1) -> Latch1/2(in_2)
  Latch1/1(out_1) -> "[bsenab]"/1
  timer dur/1 -> event timer2/2(_timer value (port))
  Latch1/2(out_2) -> Terminator/1

== system OMSv1_2/OMS v1.2  07/21/05/IM CN-LMLN/BS/FS Logic/FS Enable/FS Timing ==
  note: FS Timing
  note: * Output of TIMER circuit DISABLES output
  note: *FS Enabling is initially DISABLED
  note: Operation:
  note: * Leading Edge of input ENABLEs output
  note: (FF init state: Q=0)
  From  <= [cmpr] : Inport
  timer dur : Inport  Orientation=up  Port=2
  Latch1 : Subsystem  mask(Latch){@1=0}
      mask prompts: @1 "Initial State for Output "Q":"
      mask help: Latch
      mask init:
      | ini=(@1~=0);
      mask Help: Latches the S input.  When S (set) is one, the Q output  becomes one.  The output remains one until the R (reset) input becomes one, forcing the output to zero.  If both R and S are one, the latch will be in an undefined state.
      mask Display: disp('S   Q\n\nR  !Q')
  Terminator : Terminator
  event timer2 : Subsystem
      mask Display: disp('Event\nTimer2')
  leading edge detect : Subsystem
      mask Display: disp('Leading\nEdge Det')
  "[fsenab]" : Outport  InitialOutput=0
  wires:
  timer dur/1 -> event timer2/2(_timer value (port))
  Latch1/1(out_1) -> "[fsenab]"/1
  event timer2/1(out_1) -> Latch1/2(in_2)
  leading edge detect/1(out_1) -> Latch1/1(in_1)
  From  <= [cmpr]/1 -> event timer2/1(_PG), leading edge detect/1(in_1)
  Latch1/2(out_2) -> Terminator/1

== system OMSv1_2/OMS v1.2  07/21/05/IM CN-LMLN/BS/FS Logic/FS Enable/SampHold?1 ==
  note: When "S/H?" is LOW, then "Input" is switched directly to the
      | output ("sample").  When "S/H?" is HIGH, the current output is
      | maintained ("hold").
  Input : Inport
  S/H? : Inport  Port=2
  Memory : Memory  Orientation=left
  Sign : Subsystem
      mask Type: Sign
      mask Description: y = sign(x)
      mask Help: Sign Function:\n\t\t\ty = 1 if x > 0\n\t\t\ty = 0 if x = 0\n\t\t\ty = -1 if x < 0
      mask Display: plot(-50,-50,50,50,[-50,50],[0,0],[0,0],[-50,50],[-40,0],[-30,-30],[0,40],[30,30])
  Switch2 : Switch  Threshold=0.5  SaturateOnIntegerOverflow=on  InputSameDT=on
  output : Outport  InitialOutput=0
  wires:
  Input/1 -> Switch2/3
  Memory/1 -> Switch2/1
  S/H?/1 -> Sign/1(in_1)
  Sign/1(out_1) -> Switch2/2
  Switch2/1 -> output/1, Memory/1

== system OMSv1_2/OMS v1.2  07/21/05/IM CN-LMLN/BS/FS Logic/FS or BS?/Boolify ==
  In1 : Inport
  Abs2 : Abs  SaturateOnIntegerOverflow=on
  direction1 : Subsystem
      mask Type: Sign
      mask Description: y = sign(x)
      mask Help: Sign Function:\n\t\t\ty = 1 if x > 0\n\t\t\ty = 0 if x = 0\n\t\t\ty = -1 if x < 0
      mask Display: plot(-50,-50,50,50,[-50,50],[0,0],[0,0],[-50,50],[-40,0],[-30,-30],[0,40],[30,30])
  Out1 : Outport  InitialOutput=0
  wires:
  Abs2/1 -> direction1/1(in_1)
  In1/1 -> Abs2/1
  direction1/1(out_1) -> Out1/1

== system OMSv1_2/OMS v1.2  07/21/05/IM CN-LMLN/BS/FS Logic/FS or BS?/SampHold?1 ==
  note: When "S/H?" is LOW, then "Input" is switched directly to the
      | output ("sample").  When "S/H?" is HIGH, the current output is
      | maintained ("hold").
  Input : Inport
  S/H? : Inport  Port=2
  Memory : Memory  Orientation=left
  Sign : Subsystem
      mask Type: Sign
      mask Description: y = sign(x)
      mask Help: Sign Function:\n\t\t\ty = 1 if x > 0\n\t\t\ty = 0 if x = 0\n\t\t\ty = -1 if x < 0
      mask Display: plot(-50,-50,50,50,[-50,50],[0,0],[0,0],[-50,50],[-40,0],[-30,-30],[0,40],[30,30])
  Switch2 : Switch  Threshold=0.5  SaturateOnIntegerOverflow=on  InputSameDT=on
  output : Outport  InitialOutput=0
  wires:
  Input/1 -> Switch2/3
  Memory/1 -> Switch2/1
  S/H?/1 -> Sign/1(in_1)
  Sign/1(out_1) -> Switch2/2
  Switch2/1 -> output/1, Memory/1

== system OMSv1_2/OMS v1.2  07/21/05/IM CN-LMLN/BS/FS Logic/TCHNG Override/Latch1 ==
  in_1 : Inport
  in_2 : Inport  Port=2
  Demux : Demux  Outputs=2
  Logic : CombinatorialLogic  TruthTable=[0 1;0 1;1 0;0 1;1 0;0 1;1 0;1 0]
  Memory : Memory  Orientation=left  X0=ini
  Mux : Mux  Inputs=3
  out_1 : Outport  InitialOutput=0
  out_2 : Outport  Port=2  InitialOutput=0
  wires:
  in_2/1 -> Mux/3
  in_1/1 -> Mux/2
  Memory/1 -> Mux/1
  Demux/1 -> Memory/1, out_1/1
  Mux/1 -> Logic/1
  Logic/1 -> Demux/1
  Demux/2 -> out_2/1
